simulink model "paramServerGetterTemplate"  (R2017b)
settings: Solver=VariableStepAuto  StartTime=0.0  StopTime=inf  RelTol=1e-3
PreLoadFcn:
  | % ROS setup
  | rosshutdown;
  | ipAddr = '';
  | rosinit(ipAddr)
  | 
  | % Sample times
  | sampleTime = 0.2;
  | 
  | % Control parameters
  | ctrlParam = 2;
  | rosparam('set','/my_param',3.5);
undefined symbols (not defined in the file): X, Y
libraries: robotlib x4
settings Model: Creator=scastro  LastModifiedBy=scastro

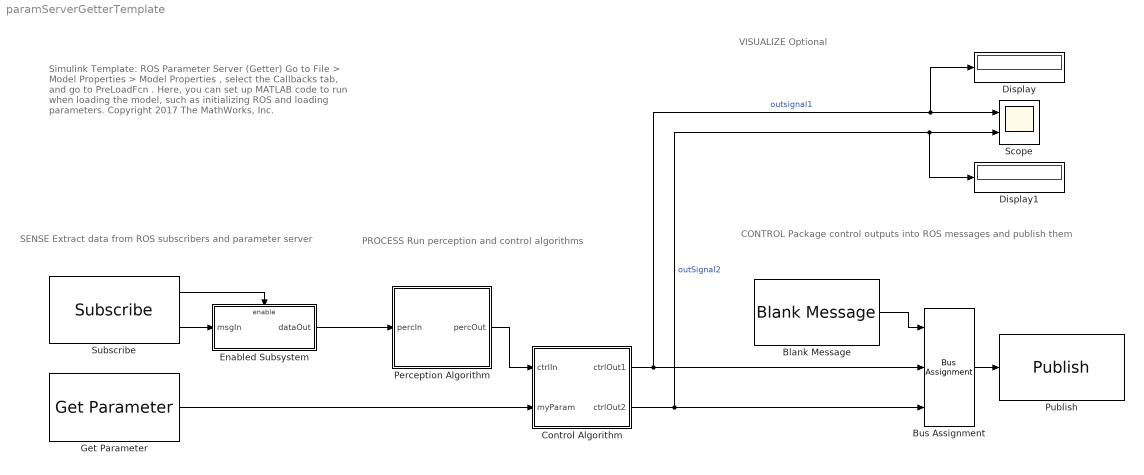
== system paramServerGetterTemplate ==
  note: Simulink Template:
      | ROS Parameter Server (Getter)
      |
      | Go to File > Model Properties > Model Properties , select the Callbacks tab, and go to PreLoadFcn .
      |
      | Here, you can set up MATLAB code to run when loading the model, such as initializing ROS and loading parameters.
      |
      | Copyright 2017 The MathWorks, Inc.
  note: PROCESS
      | Run perception and control algorithms
  note: SENSE
      | Extract data from ROS subscribers and parameter server
  note: VISUALIZE
      | Optional
  note: CONTROL
      | Package control outputs into ROS messages and publish them
  Blank Message : robotlib/Blank Message  SourceLibraryInfo=This block requires Robotics System Toolbox  messageType=geometry_msgs/Point  SampleTime=inf
      settings: SourceProductBaseCode=RO
  Bus Assignment : BusAssignment  AssignedSignals=X,Y
  Control Algorithm : Subsystem
  Display : Display
  Display1 : Display
  Enabled Subsystem : Subsystem  TreatAsAtomicUnit=on
  Get Parameter : robotlib/Get Parameter  SourceLibraryInfo=This block requires Robotics System Toolbox  ParameterSource=Select from ROS network  ParameterName=/my_param  ParameterType=double  ParameterMaxArrayLength=16  ParameterInitialValue=0.0  SampleTime=-1  ShowErrorCodeOutput=off  ModelName=paramServerGetterTemplate  BlockId=ParamGet_paramServerGetterTemplate_138
      settings: SourceProductName=Robotics System Toolbox  SourceProductBaseCode=RO
  Perception Algorithm : Subsystem
  Publish : robotlib/Publish  SourceLibraryInfo=This block requires Robotics System Toolbox  topicSource=Specify your own  topic=/my_pub_topic  messageType=geometry_msgs/Point  messageQueueLength=1
      settings: SourceProductBaseCode=RO
  Scope : Scope  NumInputPorts=2
  Subscribe : robotlib/Subscribe  SourceLibraryInfo=This block requires Robotics System Toolbox  topicSource=Select from ROS network  topic=/my_sub_topic  messageType=geometry_msgs/Point  sampleTime=-1  messageQueueLength=1
      settings: SourceProductBaseCode=RO
  wires:
  Enabled Subsystem/1(dataOut) -> Perception Algorithm/1(percIn)
  Subscribe/2 -> Enabled Subsystem/1(msgIn)
  Subscribe/1 -> Enabled Subsystem/Enable
  Bus Assignment/1 -> Publish/1
  Blank Message/1 -> Bus Assignment/1
  Perception Algorithm/1(percOut) -> Control Algorithm/1(ctrlIn)
  Control Algorithm/1(ctrlOut1) -> Display/1, Scope/1, Bus Assignment/2  "outsignal1"
  Control Algorithm/2(ctrlOut2) -> Display1/1, Scope/2, Bus Assignment/3  "outSignal2"
  Get Parameter/1 -> Control Algorithm/2(myParam)

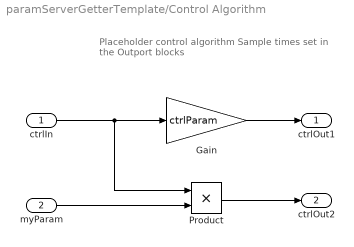
== system paramServerGetterTemplate/Control Algorithm ==
  note: Placeholder control algorithm
      |
      | Sample times set in the Outport blocks
  ctrlIn : Inport
  myParam : Inport  Port=2
  Gain : Gain  Gain=ctrlParam
  Product : Product
  ctrlOut1 : Outport  SampleTime=sampleTime
      settings: AttributesFormatString=Sample time: %<SampleTime>
  ctrlOut2 : Outport  Port=2  SampleTime=sampleTime
      settings: AttributesFormatString=Sample time: %<SampleTime>
  wires:
  ctrlIn/1 -> Product/1, Gain/1
  myParam/1 -> Product/2
  Product/1 -> ctrlOut2/1
  Gain/1 -> ctrlOut1/1

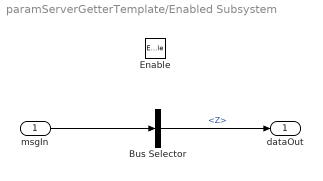
== system paramServerGetterTemplate/Enabled Subsystem ==
  msgIn : Inport
  Enable : EnablePort
  Bus Selector : BusSelector  OutputSignals=Z
  dataOut : Outport
  wires:
  msgIn/1 -> Bus Selector/1
  Bus Selector/1 -> dataOut/1  "<Z>"

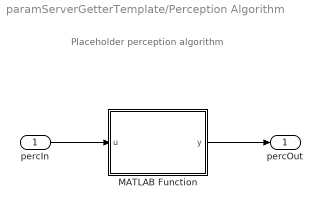
== system paramServerGetterTemplate/Perception Algorithm ==
  note: Placeholder perception algorithm
  percIn : Inport
  MATLAB Function : MATLAB Function  TreatAsAtomicUnit=on
  percOut : Outport
  wires:
  percIn/1 -> MATLAB Function/1(u)
  MATLAB Function/1(y) -> percOut/1

== matlab function paramServerGetterTemplate/Perception Algorithm/MATLAB Function ==
  data: u input; y output
function y = myPerceptionFcn(u)

y = 2*u;
